simulink library "SCAN"  (R2016a)
settings: Solver=ode45  StartTime=0.0  StopTime=10.0  RelTol=1e-3
undefined symbols (not defined in the file): CAL_FilterBufferSize, CAL_ROBO_LENG
settings Model: Creator=oelkawok  LastModifiedBy=oelkawok
settings DataIOCC: LimitDataPoints=on
settings DebuggingCC: AllowSymbolicDim=off

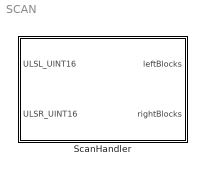
== system SCAN ==
  ScanHandler : Subsystem

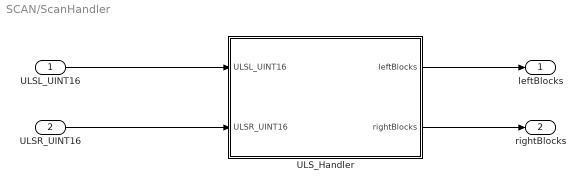
== system SCAN/ScanHandler ==
  ULSL_UINT16 : Inport  OutDataTypeStr=uint16  PortDimensions=1  SampleTime=[0.0050000000000000001,0]
  ULSR_UINT16 : Inport  Port=2  OutDataTypeStr=uint16  PortDimensions=1  SampleTime=[0.0050000000000000001,0]
  ULS_Handler : Subsystem
  leftBlocks : Outport
  rightBlocks : Outport  Port=2
  wires:
  ULSL_UINT16/1 -> ULS_Handler/1(ULSL_UINT16)
  ULSR_UINT16/1 -> ULS_Handler/2(ULSR_UINT16)
  ULS_Handler/1(leftBlocks) -> leftBlocks/1
  ULS_Handler/2(rightBlocks) -> rightBlocks/1

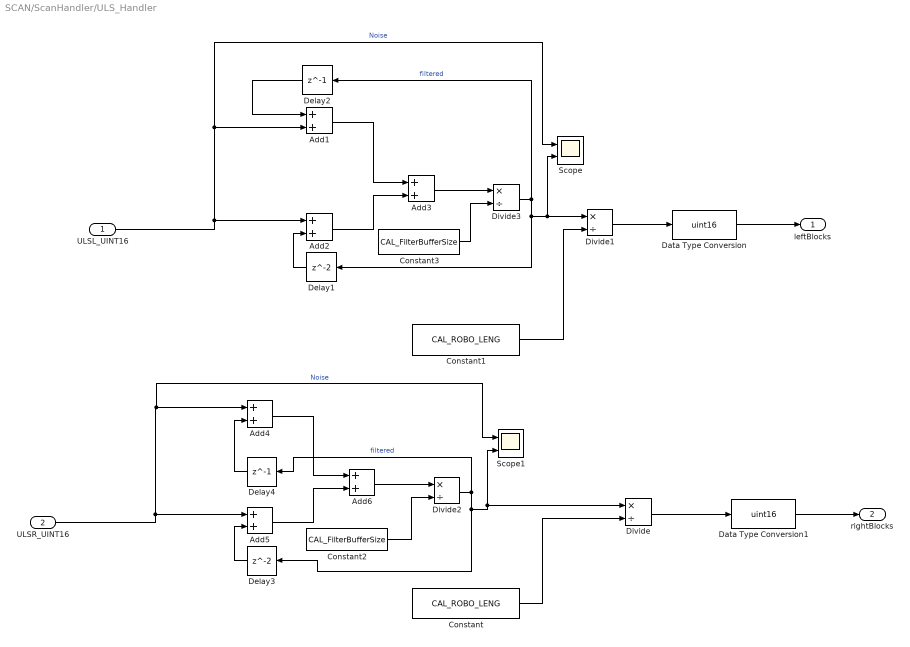
== system SCAN/ScanHandler/ULS_Handler ==
  ULSL_UINT16 : Inport  OutDataTypeStr=uint16  PortDimensions=1  SampleTime=[0.0050000000000000001,0]
  ULSR_UINT16 : Inport  Port=2  OutDataTypeStr=uint16  PortDimensions=1  SampleTime=[0.0050000000000000001,0]
  Add{1..6} (6 alike) : Sum
  Constant : Constant  Value=CAL_ROBO_LENG
  Constant1 : Constant  Value=CAL_ROBO_LENG
  Constant2 : Constant  Value=CAL_FilterBufferSize  OutDataTypeStr=Inherit: Inherit via back propagation
  Constant3 : Constant  Value=CAL_FilterBufferSize  OutDataTypeStr=Inherit: Inherit via back propagation
  Data Type Conversion : DataTypeConversion  OutDataTypeStr=uint16
  Data Type Conversion1 : DataTypeConversion  OutDataTypeStr=uint16
  Delay1 : Delay  InitialCondition=0
  Delay2 : Delay  DelayLength=1  InitialCondition=0
  Delay3 : Delay  InitialCondition=0
  Delay4 : Delay  DelayLength=1  InitialCondition=0
  Divide{,1..3} (4 alike) : Product  Inputs=*/
  Scope : Scope  NumInputPorts=2
  Scope1 : Scope  NumInputPorts=2
  leftBlocks : Outport
  rightBlocks : Outport  Port=2
  wires:
  Divide2/1 -> Delay4/1, Delay3/1, Divide/1, Scope1/2  "filtered"
  Constant2/1 -> Divide2/2
  Add6/1 -> Divide2/1
  Add5/1 -> Add6/2
  Add4/1 -> Add6/1
  Delay3/1 -> Add5/2
  ULSR_UINT16/1 -> Add5/1, Add4/1, Scope1/1  "Noise"
  Delay4/1 -> Add4/2
  Divide3/1 -> Delay2/1, Delay1/1, Divide1/1, Scope/2  "filtered"
  Constant3/1 -> Divide3/2
  Add3/1 -> Divide3/1
  Add2/1 -> Add3/2
  Add1/1 -> Add3/1
  Delay1/1 -> Add2/2
  ULSL_UINT16/1 -> Add2/1, Scope/1, Add1/2  "Noise"
  Delay2/1 -> Add1/1
  Constant/1 -> Divide/2
  Constant1/1 -> Divide1/2
  Divide/1 -> Data Type Conversion1/1
  Divide1/1 -> Data Type Conversion/1
  Data Type Conversion/1 -> leftBlocks/1
  Data Type Conversion1/1 -> rightBlocks/1
